simulink library "revenue_module"  (R2025b)
settings: Solver=VariableStepAuto  StartTime=0.0  StopTime=10.0  RelTol=1e-3
settings Model: Creator=ciepm  LastModifiedBy=ciepm

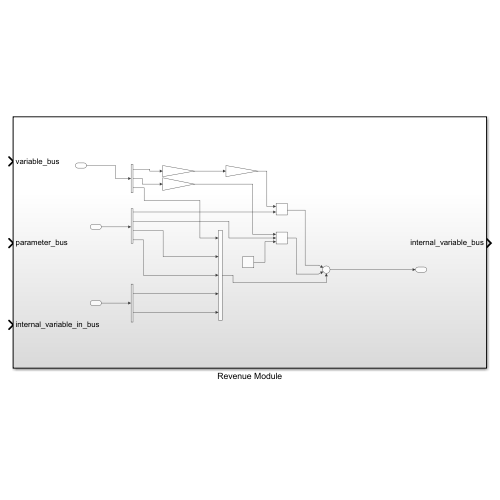
[thumbnail: Simulink's stored preview of the top-level diagram]
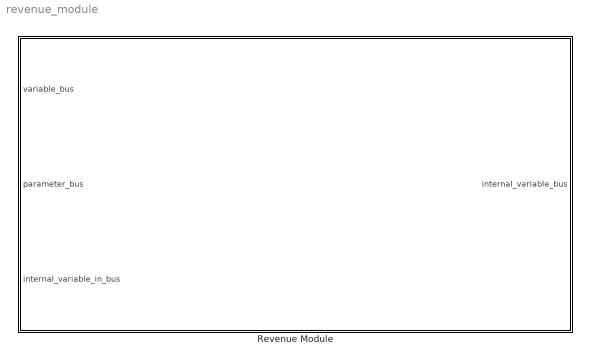
== system revenue_module ==
  Revenue Module : Subsystem

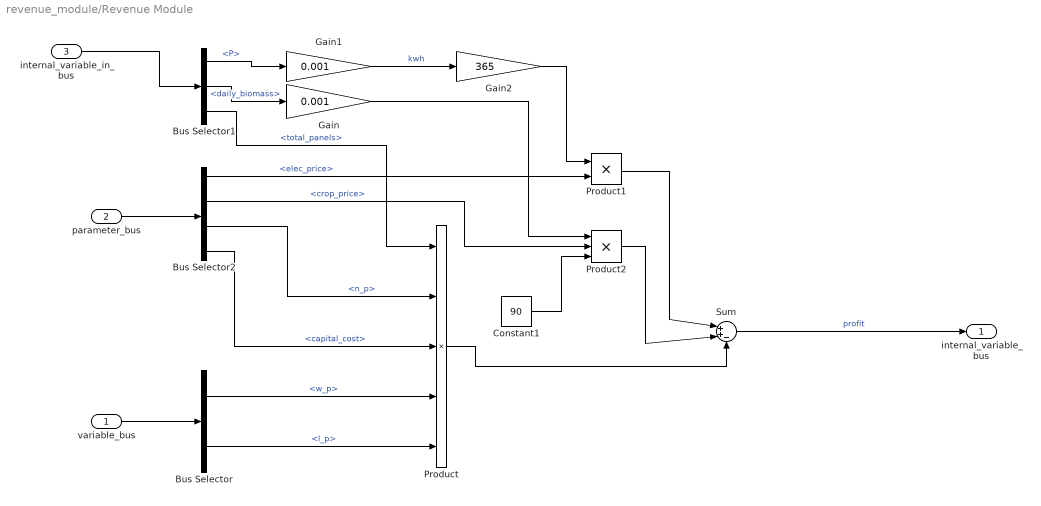
== system revenue_module/Revenue Module ==
  variable_bus : Inport
  parameter_bus : Inport  Port=2
  internal_variable_in_bus : Inport  Port=3
  Bus Selector : BusSelector  OutputSignals=PV.w_p,PV.l_p
  Bus Selector1 : BusSelector  OutputSignals=energy_per_day.P,daily_biomass,energy_per_day.total_panels
  Bus Selector2 : BusSelector  OutputSignals=crop.elec_price,crop.crop_price,PV.n_p,crop.capital_cost
  Constant1 : Constant  Value=90
  Gain : Gain  Gain=0.001
  Gain1 : Gain  Gain=0.001
  Gain2 : Gain  Gain=365
  Product : Product  Inputs=5
  Product1 : Product
  Product2 : Product  Inputs=3
  Sum : Sum  Inputs=|++-
  internal_variable_bus : Outport
  wires:
  Bus Selector1/3 -> Product/1  "<total_panels>"
  Bus Selector/2 -> Product/5  "<l_p>"
  Bus Selector/1 -> Product/4  "<w_p>"
  Bus Selector2/4 -> Product/3  "<capital_cost>"
  Bus Selector2/3 -> Product/2  "<n_p>"
  Gain2/1 -> Product1/1
  Gain1/1 -> Gain2/1  "kwh"
  Bus Selector1/1 -> Gain1/1  "<P>"
  Gain/1 -> Product2/1
  Bus Selector1/2 -> Gain/1  "<daily_biomass>"
  Constant1/1 -> Product2/3
  Product2/1 -> Sum/2
  Product1/1 -> Sum/1
  Bus Selector2/2 -> Product2/2  "<crop_price>"
  Bus Selector2/1 -> Product1/2  "<elec_price>"
  Product/1 -> Sum/3
  internal_variable_in_bus/1 -> Bus Selector1/1
  parameter_bus/1 -> Bus Selector2/1
  variable_bus/1 -> Bus Selector/1
  Sum/1 -> internal_variable_bus/1  "profit"
